simulink model "QuadcopterSimulation"  (R2023b)
settings: Solver=FixedStepAuto  StartTime=0.0  StopTime=180  FixedStep=SampleTime  RelTol=1e-3
PreLoadFcn:
  | %Based on the quadcopter model used in jMAVSim
  | 
  | Ixx = 0.005; %Kgm^2
  | Iyy = 0.005;
  | Izz = 0.009;
  | 
  | 
  | inertia = diag([Ixx, Iyy, Izz]);
  | 
  | mass = 0.8; %Kg
  | g = 9.81; %m/s^2
  | 
  | armLength = 0.33/2; % length of Arm measured from center in m
  | 
  | rotorThrustMax = 4; %N
  | 
  | rotorTorqueMax = 0.05 %Nm
  | 
  | rotorTimeConst = 0.005 % time constant of rotor (motor + propeller)
  | 
  | %rotorOffset = [0 0 0]; % Rotors position offsets from Gravity center
  | 
  | dragCoeffMov = 0.01; %drag coefficient for linear motion of quadcopter
  | 
  | % Initial states
  | init.posNED = [0, 0, 0]; % m
  | init.vb = [0 0 0]'; %m/s
  | init.euler = [0, 0, 0]'; %Roll Pitch Yaw Rads
  | init.angRates = [0, 0, 0]; %rad/s
  | 
  | 
  | %Computed from above values
  | rotorPositions = zeros(3,4);
  | axisD = armLength/sqrt(2);
  | rotorPositions(:,1) = [axisD, axisD, 0]';
  | rotorPositions(:,2) = [-axisD, -axisD, 0]';
  | rotorPositions(:,3) = [+axisD, -axisD, 0]';
  | rotorPositions(:,4) = [-axisD, axisD, 0]';
  | rotorDir = [-1, -1, 1, 1]; %rotation direction. +ve = clockwise
undefined symbols (not defined in the file): ax, ay, az, Earth, Payload, SampleTime, vx, vy, vz, WGS84, windVel, x, y, z
libraries: px4uORBlib x2, aerolibtransform2 x1, uavmavlinklib x1
settings Model: Creator=The MathWorks, Inc.  LastModifiedBy=LonelyRetard420
settings SolverCC: AlgebraicLoopSolver=LineSearch
settings DebuggingCC: AlgebraicLoopMsg=none  UnconnectedInputMsg=warning  UnconnectedOutputMsg=warning  UnconnectedLineMsg=warning
settings ModelReferenceCC: EnableRefExpFcnMdlSchedulingChecks=on
settings RTWCC: DLArmComputeVersion=19.05

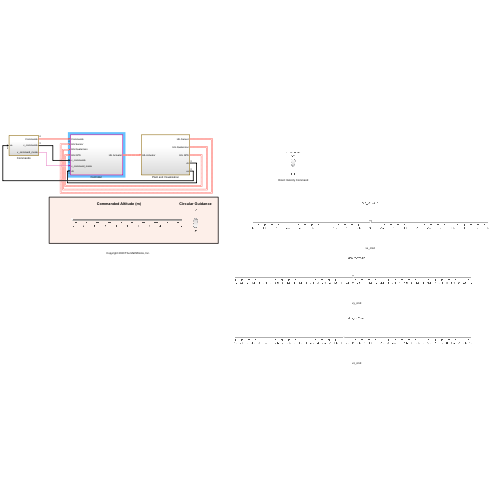
[thumbnail: Simulink's stored preview of the top-level diagram]
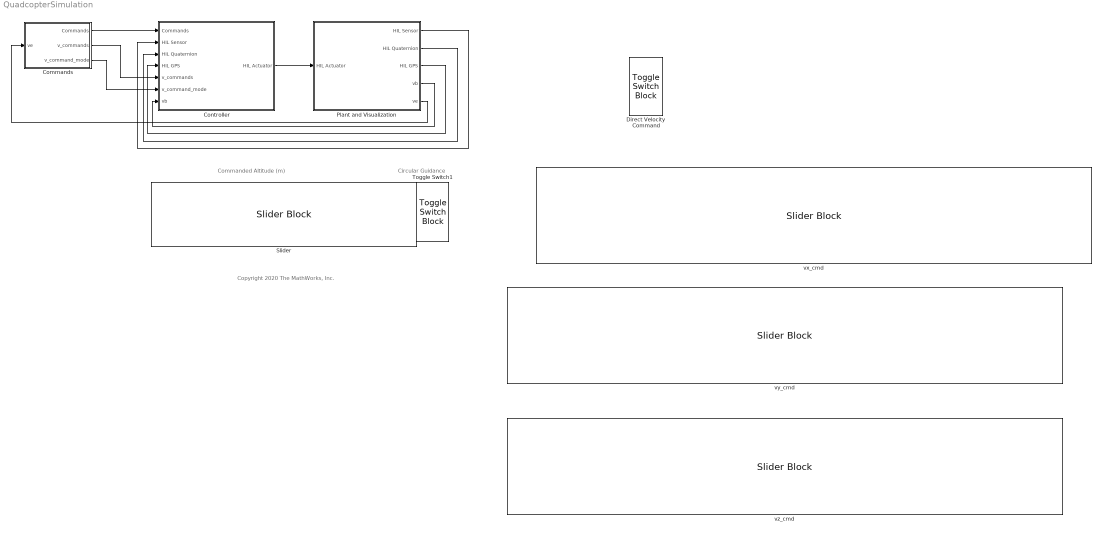
== system QuadcopterSimulation ==
  note: Commanded Altitude (m)
  note: Circular Guidance
  note: Copyright 2020 The MathWorks, Inc.
  Commands : Subsystem
  "Controller " : Subsystem
  Direct Velocity Command : ToggleSwitchBlock
      settings: Values={{'Off', 'On'}, [0 1]}
  Plant and Visualization : Subsystem
  Slider : SliderBlock  LabelPosition=Hide  ScaleMin=-10  ScaleMax=0  TickInterval=1
  Toggle Switch1 : ToggleSwitchBlock  LabelPosition=Hide
      settings: Values={{'Off', 'On'}, [0 1]}
  vx_cmd : SliderBlock  ScaleMin=-5  ScaleMax=5  TickInterval=0.5
  vy_cmd : SliderBlock  ScaleMin=-10  ScaleMax=10  TickInterval=0.5
  vz_cmd : SliderBlock  ScaleMin=-10  ScaleMax=10  TickInterval=0.5
  wires:
  Commands/1(Commands) -> "Controller "/1(Commands)
  "Controller "/1(HIL Actuator) -> Plant and Visualization/1(HIL Actuator)
  Plant and Visualization/1(HIL Sensor) -> "Controller "/2(HIL Sensor)
  Plant and Visualization/2(HIL Quaternion) -> "Controller "/3(HIL Quaternion)
  Plant and Visualization/3(HIL GPS) -> "Controller "/4(HIL GPS)
  Commands/2(v_commands) -> "Controller "/5(v_commands)
  Commands/3(v_command_mode) -> "Controller "/6(v_command_mode)
  Plant and Visualization/4(vb) -> "Controller "/7(vb)
  Plant and Visualization/5(ve) -> Commands/1(ve)

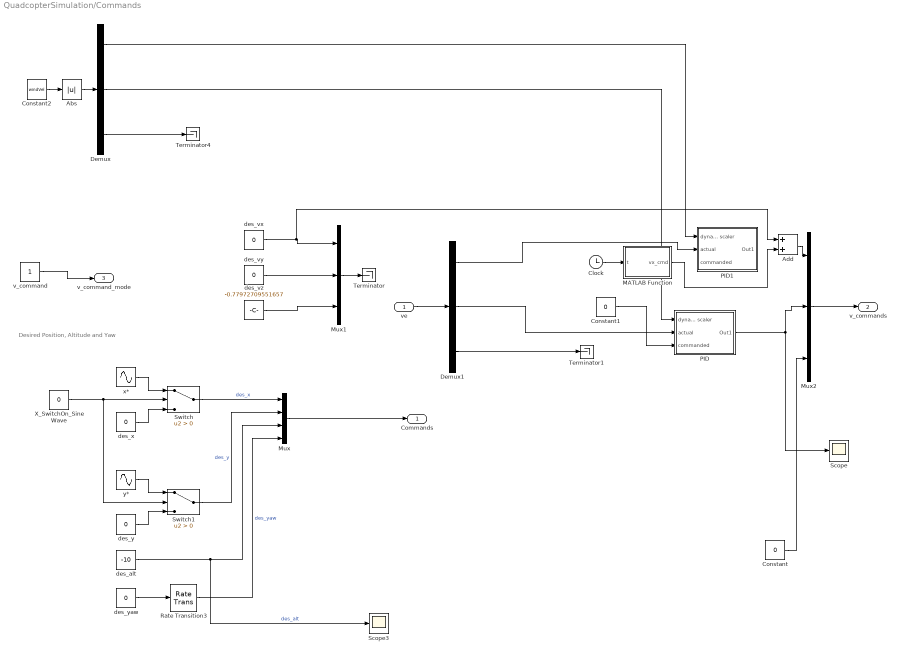
== system QuadcopterSimulation/Commands ==
  note: Desired Position, Altitude and Yaw
  ve : Inport
  Abs : Abs  SaturateOnIntegerOverflow=off
  Add : Sum
  Clock : Clock
  Constant : Constant  Value=0
  Constant1 : Constant  Value=0
  Constant2 : Constant  Value=windVel
  Demux : Demux  Outputs=3
  Demux1 : Demux  Outputs=3
  MATLAB Function : MATLAB Function  TreatAsAtomicUnit=on
  Mux : Mux
  Mux1 : Mux  Inputs=3
  Mux2 : Mux  Inputs=3
  PID : Subsystem
  PID1 : Subsystem
  Rate Transition3 : RateTransition  OutPortSampleTime=SampleTime
  Scope : Scope
  Scope3 : Scope
  Switch : Switch  Criteria=u2 > Threshold  SaturateOnIntegerOverflow=off  InputSameDT=off
  Switch1 : Switch  Criteria=u2 > Threshold  SaturateOnIntegerOverflow=off  InputSameDT=off
  Terminator : Terminator
  Terminator1 : Terminator
  Terminator4 : Terminator
  X_SwitchOn_Sine Wave : Constant  Value=0  SampleTime=SampleTime
  des_alt : Constant  Value=-10  SampleTime=SampleTime
  des_vx : Constant  Value=0
  des_vy : Constant  Value=0
  des_vz : Constant  Value=-0.77972709551657
  des_x : Constant  Value=0  SampleTime=SampleTime
  des_y : Constant  Value=0  SampleTime=SampleTime
  des_yaw : Constant  Value=0  SampleTime=SampleTime
  v_command : Constant
  x* : Sin  Frequency=2*pi*.125  Phase=-pi/2  Samples=10000  SampleTime=SampleTime
  y* : Sin  Frequency=2*pi*.125  Samples=10000  SampleTime=SampleTime
  Commands : Outport
  v_commands : Outport  Port=2
  v_command_mode : Outport  Port=3
  wires:
  Rate Transition3/1 -> Mux/4  "des_yaw"
  des_x/1 -> Switch/3
  Switch/1 -> Mux/1  "des_x"
  Switch1/1 -> Mux/2  "des_y"
  X_SwitchOn_Sine Wave/1 -> Switch1/2, Switch/2
  des_yaw/1 -> Rate Transition3/1
  y*/1 -> Switch1/1
  des_y/1 -> Switch1/3
  x*/1 -> Switch/1
  des_alt/1 -> Scope3/1, Mux/3  "des_alt"
  des_vy/1 -> Mux1/2
  des_vz/1 -> Mux1/3
  des_vx/1 -> Add/1, Mux1/1
  Mux/1 -> Commands/1
  Mux1/1 -> Terminator/1
  v_command/1 -> v_command_mode/1
  Mux2/1 -> v_commands/1
  Clock/1 -> MATLAB Function/1(t)
  Constant2/1 -> Abs/1
  Abs/1 -> Demux/1
  ve/1 -> Demux1/1
  Demux1/3 -> Terminator1/1
  Constant/1 -> Mux2/3
  Demux1/1 -> PID1/2(actual)
  Demux/3 -> Terminator4/1
  PID/1(Out1) -> Mux2/2, Scope/1
  Demux/2 -> PID/1(dynamic gain scaler)
  Demux1/2 -> PID/2(actual)
  Constant1/1 -> PID/3(commanded)
  Demux/1 -> PID1/1(dynamic gain scaler)
  Add/1 -> Mux2/1
  MATLAB Function/1(vx_cmd) -> Add/2

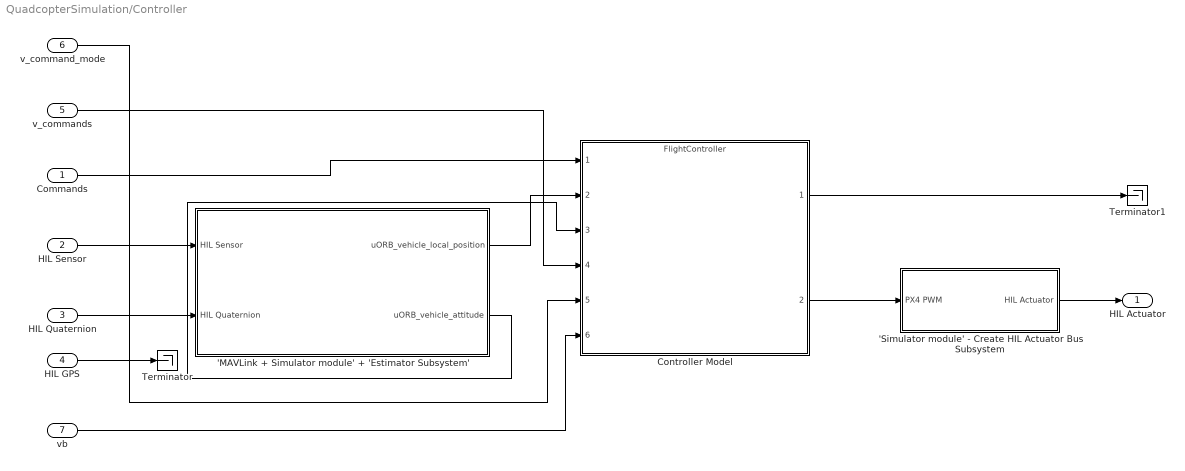
== system QuadcopterSimulation/Controller  ==
  Commands : Inport
  HIL Sensor : Inport  Port=2
  HIL Quaternion : Inport  Port=3
  HIL GPS : Inport  Port=4
  v_commands : Inport  Port=5
  v_command_mode : Inport  Port=6
  vb : Inport  Port=7
  'MAVLink + Simulator module' + 'Estimator Subsystem' : Subsystem
      settings: PortSchema="{\"entries\":[{\"content\":{\"sides\":[{\"content\":{\"connectorIds\":[]},\"type\":\"ConnectorPlacement.EquallySpacedRectSide\",\"uuid\":\"18f19b7f-7de0-4ac4-a24f-d8ceb747f924\"},{\"content\":{\"connectorIds\":[],\"side\":\"RIGHT\"},\"type\":\"ConnectorPlacement.EquallySpacedRectSide\",\"uuid\":\"b474fbae-f8e2-4c2b-be96-a63ee47992dd\"},{\"content\":{\"connectorIds\":[\"In1\",\"In2\"],\"side\":\"TOP\"},\"type\":\"ConnectorPlacement.EquallySpacedRectSide\",\"uuid\":\"67540526-de5d-4152-a323-fd05419e6390\"},{\"content\":{\"connectorIds\":[\"Out1\",\"Out2\"],\"side\":\"BOTTOM\"},\"type\":\"ConnectorPlacement.EquallySpacedRectSide\",\"uuid\":\"c51ef1bd-db79-4835-87f1-e9dccd8fce9f\"},{\"content\":{\"connectorIds\":[],\"side\":\"HIDDEN\"},\"type\":\"ConnectorPlacement.EquallySpacedRectSide\",\"uuid\":\"82a3913e-38ee-407a-aef4-9df458d840d7\"}]},\"type\":\"ConnectorPlacement.EquallySpacedConnector\",\"uuid\":\"5015a705-00cf-433b-8716-d3e1ebe8eda0\"}],\"packageUris\":[\"http://schema.mathworks.com/mf0/Connector/R2020b\"],\"version\":\"1.0\"}"
  'Simulator module' - Create HIL Actuator Bus Subsystem : Subsystem
  Controller Model : ModelReference  ModelNameDialog=FlightController.slx  SimulationMode=Normal  ModelReferenceVersion=7.7
  Terminator : Terminator
  Terminator1 : Terminator
  HIL Actuator : Outport
  wires:
  Controller Model/2 -> 'Simulator module' - Create HIL Actuator Bus Subsystem/1(PX4 PWM)
  'Simulator module' - Create HIL Actuator Bus Subsystem/1(HIL Actuator) -> HIL Actuator/1
  HIL Sensor/1 -> 'MAVLink + Simulator module' + 'Estimator Subsystem'/2(HIL Sensor)
  HIL Quaternion/1 -> 'MAVLink + Simulator module' + 'Estimator Subsystem'/1(HIL Quaternion)
  Commands/1 -> Controller Model/1
  'MAVLink + Simulator module' + 'Estimator Subsystem'/2(uORB_vehicle_local_position) -> Controller Model/2
  'MAVLink + Simulator module' + 'Estimator Subsystem'/1(uORB_vehicle_attitude) -> Controller Model/3
  HIL GPS/1 -> Terminator/1
  Controller Model/1 -> Terminator1/1
  v_commands/1 -> Controller Model/4
  v_command_mode/1 -> Controller Model/5
  vb/1 -> Controller Model/6

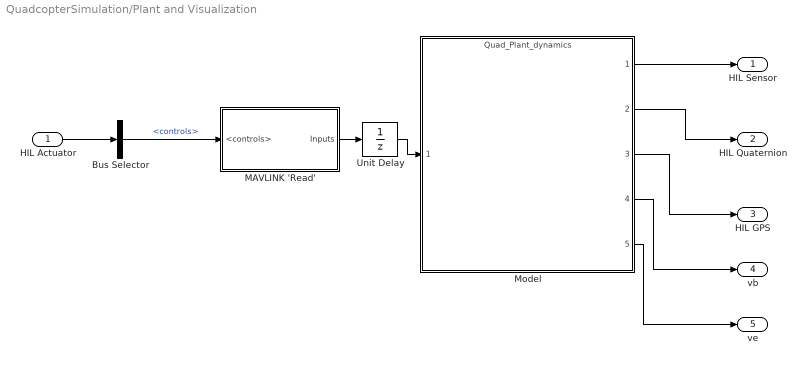
== system QuadcopterSimulation/Plant and Visualization ==
  HIL Actuator : Inport
  Bus Selector : BusSelector  OutputSignals=Payload.controls
  MAVLINK 'Read' : Subsystem
  Model : ModelReference  ModelNameDialog=Quad_Plant_dynamics.slx  SimulationMode=Normal  ModelReferenceVersion=7.29
  Unit Delay : UnitDelay  InitialCondition=[0 0 0 0]  SampleTime=-1  HasFrameUpgradeWarning=on
  HIL Sensor : Outport
  HIL Quaternion : Outport  Port=2
  HIL GPS : Outport  Port=3
  vb : Outport  Port=4
  ve : Outport  Port=5
  wires:
  HIL Actuator/1 -> Bus Selector/1
  Bus Selector/1 -> MAVLINK 'Read'/1(<controls>)  "<controls>"
  MAVLINK 'Read'/1(Inputs) -> Unit Delay/1
  Model/1 -> HIL Sensor/1
  Model/2 -> HIL Quaternion/1
  Model/3 -> HIL GPS/1
  Unit Delay/1 -> Model/1
  Model/4 -> vb/1
  Model/5 -> ve/1

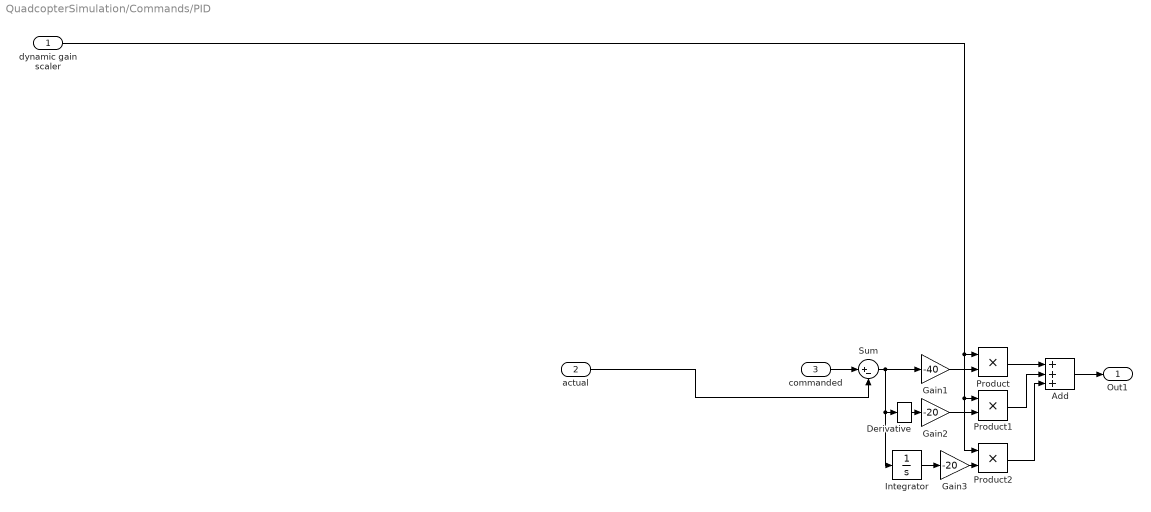
== system QuadcopterSimulation/Commands/PID ==
  dynamic gain scaler : Inport
  actual : Inport  Port=2
  commanded : Inport  Port=3
  Add : Sum  Inputs=+++
  Derivative : Derivative
  Gain1 : Gain  Gain=-40
  Gain2 : Gain  Gain=-20
  Gain3 : Gain  Gain=-20
  Integrator : Integrator
  Product : Product
  Product1 : Product
  Product2 : Product
  Sum : Sum  Inputs=|+-
  Out1 : Outport
  wires:
  Gain1/1 -> Product/2
  Integrator/1 -> Gain3/1
  Sum/1 -> Integrator/1, Derivative/1, Gain1/1
  Product/1 -> Add/1
  Product2/1 -> Add/3
  Gain2/1 -> Product1/2
  dynamic gain scaler/1 -> Product2/1, Product1/1, Product/1
  Product1/1 -> Add/2
  Gain3/1 -> Product2/2
  actual/1 -> Sum/2
  Derivative/1 -> Gain2/1
  Add/1 -> Out1/1
  commanded/1 -> Sum/1

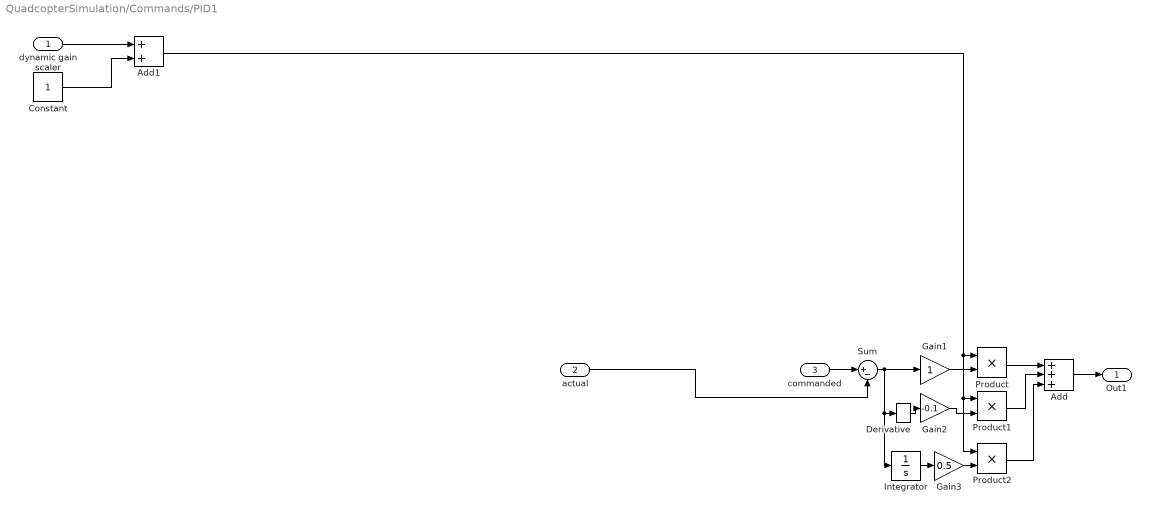
== system QuadcopterSimulation/Commands/PID1 ==
  dynamic gain scaler : Inport
  actual : Inport  Port=2
  commanded : Inport  Port=3
  Add : Sum  Inputs=+++
  Add1 : Sum
  Constant : Constant
  Derivative : Derivative
  Gain1 : Gain
  Gain2 : Gain  Gain=-0.1
  Gain3 : Gain  Gain=0.5
  Integrator : Integrator
  Product : Product
  Product1 : Product
  Product2 : Product
  Sum : Sum  Inputs=|+-
  Out1 : Outport
  wires:
  Gain1/1 -> Product/2
  Integrator/1 -> Gain3/1
  Sum/1 -> Integrator/1, Derivative/1, Gain1/1
  Product/1 -> Add/1
  Product2/1 -> Add/3
  Gain2/1 -> Product1/2
  Product1/1 -> Add/2
  Gain3/1 -> Product2/2
  actual/1 -> Sum/2
  Derivative/1 -> Gain2/1
  Add/1 -> Out1/1
  commanded/1 -> Sum/1
  Add1/1 -> Product2/1, Product1/1, Product/1
  dynamic gain scaler/1 -> Add1/1
  Constant/1 -> Add1/2

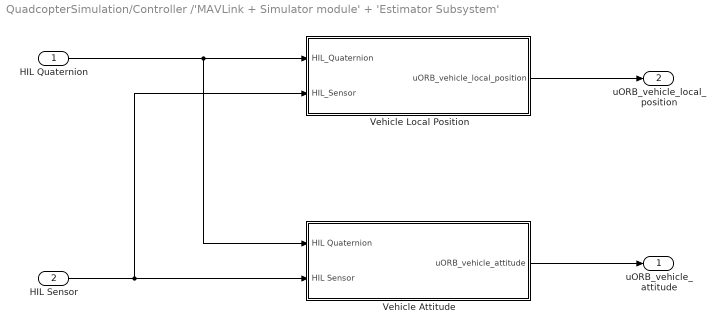
== system QuadcopterSimulation/Controller /'MAVLink + Simulator module' + 'Estimator Subsystem' ==
  HIL Quaternion : Inport
  HIL Sensor : Inport  Port=2
  Vehicle Attitude : Subsystem
  Vehicle Local Position : Subsystem
  uORB_vehicle_attitude : Outport
  uORB_vehicle_local_position : Outport  Port=2
  wires:
  HIL Quaternion/1 -> Vehicle Attitude/1(HIL Quaternion), Vehicle Local Position/1(HIL_Quaternion)
  HIL Sensor/1 -> Vehicle Local Position/2(HIL_Sensor), Vehicle Attitude/2(HIL Sensor)
  Vehicle Local Position/1(uORB_vehicle_local_position) -> uORB_vehicle_local_position/1
  Vehicle Attitude/1(uORB_vehicle_attitude) -> uORB_vehicle_attitude/1

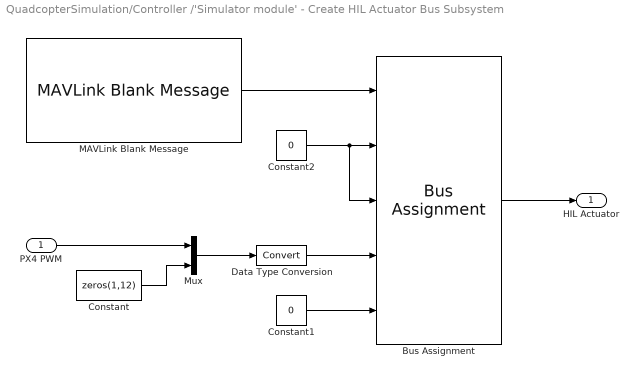
== system QuadcopterSimulation/Controller /'Simulator module' - Create HIL Actuator Bus Subsystem ==
  PX4 PWM : Inport
  Bus Assignment : BusAssignment  AssignedSignals=Payload.time_usec,Payload.flags,Payload.controls,Payload.mode
  Constant : Constant  Value=zeros(1,12)  OutDataTypeStr=Inherit: Inherit via back propagation  SampleTime=SampleTime
  Constant1 : Constant  Value=0  OutDataTypeStr=Inherit: Inherit via back propagation  SampleTime=SampleTime
  Constant2 : Constant  Value=0  OutDataTypeStr=Inherit: Inherit via back propagation  SampleTime=SampleTime
  Data Type Conversion : DataTypeConversion  SaturateOnIntegerOverflow=off  RndMeth=Floor
  MAVLink Blank Message : uavmavlinklib/MAVLink Blank Message  dialectSource=Select from standard MAVLink dialects  dialect=common.xml  dialectCustom=common.xml  version=2  messageType=HIL_ACTUATOR_CONTROLS  SystemID=1  ComponentID=1  SampleTime=SampleTime
  Mux : Mux  Inputs=2
  HIL Actuator : Outport
  wires:
  MAVLink Blank Message/1 -> Bus Assignment/1
  Bus Assignment/1 -> HIL Actuator/1
  PX4 PWM/1 -> Mux/1
  Constant/1 -> Mux/2
  Mux/1 -> Data Type Conversion/1
  Constant2/1 -> Bus Assignment/3, Bus Assignment/2
  Constant1/1 -> Bus Assignment/5
  Data Type Conversion/1 -> Bus Assignment/4

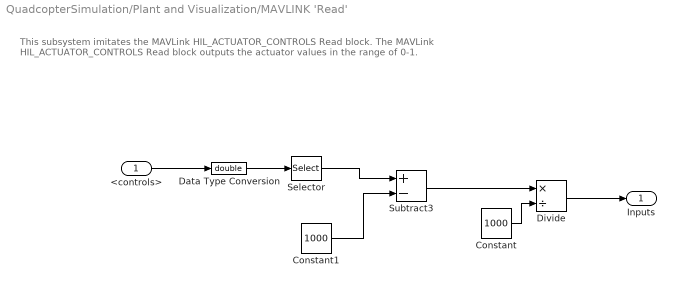
== system QuadcopterSimulation/Plant and Visualization/MAVLINK 'Read' ==
  note: This subsystem imitates the MAVLink HIL_ACTUATOR_CONTROLS Read block. The MAVLink HIL_ACTUATOR_CONTROLS Read block outputs the
      | actuator values in the range of 0-1.
  <controls> : Inport
  Constant : Constant  Value=1000  SampleTime=SampleTime
  Constant1 : Constant  Value=1000  OutDataTypeStr=Inherit: Inherit via back propagation  SampleTime=SampleTime
  Data Type Conversion : DataTypeConversion  OutDataTypeStr=double  SaturateOnIntegerOverflow=off  RndMeth=Floor
  Divide : Product  Inputs=*/
  Selector : Selector  InputPortWidth=16  IndexOptions=Index vector (dialog)  Indices=[1:4]  OutputSizes=1
  Subtract3 : Sum  Inputs=+-
  Inputs : Outport
  wires:
  <controls>/1 -> Data Type Conversion/1
  Constant/1 -> Divide/2
  Data Type Conversion/1 -> Selector/1
  Constant1/1 -> Subtract3/2
  Subtract3/1 -> Divide/1
  Selector/1 -> Subtract3/1
  Divide/1 -> Inputs/1

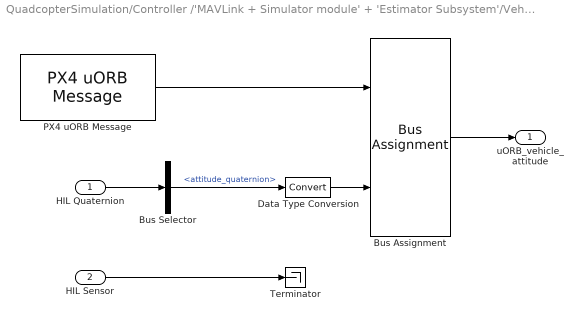
== system QuadcopterSimulation/Controller /'MAVLink + Simulator module' + 'Estimator Subsystem'/Vehicle Attitude ==
  HIL Quaternion : Inport
  HIL Sensor : Inport  Port=2
  Bus Assignment : BusAssignment  AssignedSignals=q
  Bus Selector : BusSelector  OutputSignals=Payload.attitude_quaternion
  Data Type Conversion : DataTypeConversion  SaturateOnIntegerOverflow=off  RndMeth=Floor
  PX4 uORB Message : px4uORBlib/PX4 uORB Message  uORBTopic=vehicle_attitude  SampleTime=SampleTime  selectInstance=vehicle_attitude
  Terminator : Terminator
  uORB_vehicle_attitude : Outport
  wires:
  HIL Quaternion/1 -> Bus Selector/1
  Data Type Conversion/1 -> Bus Assignment/2
  PX4 uORB Message/1 -> Bus Assignment/1
  Bus Assignment/1 -> uORB_vehicle_attitude/1
  HIL Sensor/1 -> Terminator/1
  Bus Selector/1 -> Data Type Conversion/1  "<attitude_quaternion>"

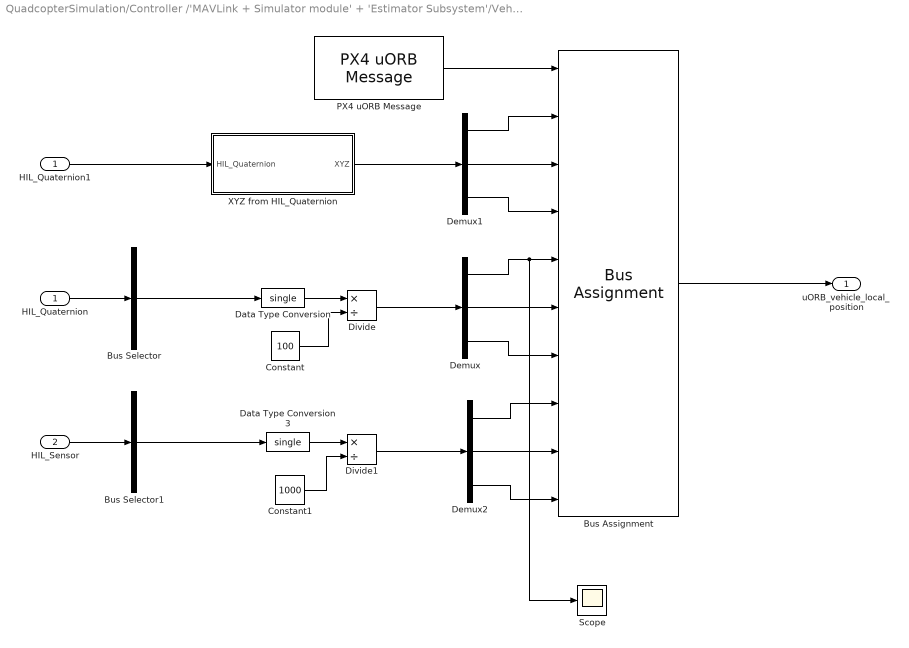
== system QuadcopterSimulation/Controller /'MAVLink + Simulator module' + 'Estimator Subsystem'/Vehicle Local Position ==
  HIL_Quaternion : Inport
  HIL_Sensor : Inport  Port=2
  Bus Assignment : BusAssignment  AssignedSignals=x,y,z,vx,vy,vz,ax,ay,az
  Bus Selector : BusSelector  OutputSignals=Payload.vx,Payload.vy,Payload.vz  OutputAsBus=on
  Bus Selector1 : BusSelector  OutputSignals=Payload.xacc,Payload.yacc,Payload.zacc  OutputAsBus=on
  Constant : Constant  Value=100  OutDataTypeStr=single  SampleTime=SampleTime
  Constant1 : Constant  Value=1000  OutDataTypeStr=single  SampleTime=SampleTime
  Data Type Conversion : DataTypeConversion  OutDataTypeStr=single  SaturateOnIntegerOverflow=off  RndMeth=Floor
  Data Type Conversion3 : DataTypeConversion  OutDataTypeStr=single  SaturateOnIntegerOverflow=off  RndMeth=Floor
  Demux : Demux  Outputs=3
  Demux1 : Demux  Outputs=3
  Demux2 : Demux  Outputs=3
  Divide : Product  Inputs=*/
  Divide1 : Product  Inputs=*/
  HIL_Quaternion1 : InportShadow
  PX4 uORB Message : px4uORBlib/PX4 uORB Message  uORBTopic=vehicle_local_position  SampleTime=SampleTime  selectInstance=vehicle_local_position
  Scope : Scope
  XYZ from HIL_Quaternion : Subsystem
  uORB_vehicle_local_position : Outport
  wires:
  Bus Assignment/1 -> uORB_vehicle_local_position/1
  PX4 uORB Message/1 -> Bus Assignment/1
  Demux/3 -> Bus Assignment/7
  Bus Selector/1 -> Data Type Conversion/1
  Demux/1 -> Scope/1, Bus Assignment/5
  Demux/2 -> Bus Assignment/6
  Demux1/3 -> Bus Assignment/4
  Demux1/1 -> Bus Assignment/2
  Demux1/2 -> Bus Assignment/3
  Data Type Conversion/1 -> Divide/1
  HIL_Quaternion/1 -> Bus Selector/1
  Divide/1 -> Demux/1
  Constant/1 -> Divide/2
  Demux2/2 -> Bus Assignment/9
  Demux2/1 -> Bus Assignment/8
  Demux2/3 -> Bus Assignment/10
  Divide1/1 -> Demux2/1
  Bus Selector1/1 -> Data Type Conversion3/1
  HIL_Sensor/1 -> Bus Selector1/1
  Data Type Conversion3/1 -> Divide1/1
  Constant1/1 -> Divide1/2
  HIL_Quaternion1/1 -> XYZ from HIL_Quaternion/1(HIL_Quaternion)
  XYZ from HIL_Quaternion/1(XYZ) -> Demux1/1

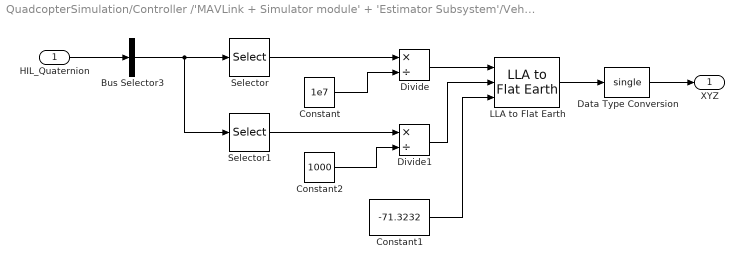
== system QuadcopterSimulation/Controller /'MAVLink + Simulator module' + 'Estimator Subsystem'/Vehicle Local Position/XYZ from HIL_Quaternion ==
  HIL_Quaternion : Inport
  Bus Selector3 : BusSelector  OutputSignals=Payload.lat,Payload.lon,Payload.alt  OutputAsBus=on
  Constant : Constant  Value=1e7  OutDataTypeStr=double
  Constant1 : Constant  Value=-71.3232  OutDataTypeStr=double
  Constant2 : Constant  Value=1000  OutDataTypeStr=double
  Data Type Conversion : DataTypeConversion  OutDataTypeStr=single  SaturateOnIntegerOverflow=off  RndMeth=Floor
  Divide : Product  Inputs=*/
  Divide1 : Product  Inputs=*/
  LLA to Flat Earth : aerolibtransform2/LLA to Flat Earth  units=Metric (MKS)  ptype=Earth (WGS84)  F=1/298.257223563  R=6378137  refPosPort=off  LL0=[0 10]  psi=0
  Selector : Selector  InputPortWidth=3  IndexOptions=Index vector (dialog)  Indices=[1:2]  OutputSizes=1
  Selector1 : Selector  InputPortWidth=3  IndexOptions=Index vector (dialog)  Indices=[3]  OutputSizes=1
  XYZ : Outport
  wires:
  HIL_Quaternion/1 -> Bus Selector3/1
  Constant1/1 -> LLA to Flat Earth/3
  Constant/1 -> Divide/2
  Bus Selector3/1 -> Selector1/1, Selector/1
  Selector/1 -> Divide/1
  Constant2/1 -> Divide1/2
  Selector1/1 -> Divide1/1
  Divide/1 -> LLA to Flat Earth/1
  Divide1/1 -> LLA to Flat Earth/2
  LLA to Flat Earth/1 -> Data Type Conversion/1
  Data Type Conversion/1 -> XYZ/1

== matlab function QuadcopterSimulation/Commands/MATLAB Function ==
  data: vx_cmd output; t input
function vx_cmd = fcn(t)
    if t<30
        vx_cmd=0;
    else 
        incrementCount=1+floor((t-30)/5);
        if (incrementCount<=30) vx_cmd=0.116666*incrementCount;
        else 
            vx_cmd=3.5;
        end
    end
